simulink model "sampleModel1577"  (R2023a)
settings: Solver=VariableStepAuto  StartTime=0.0  StopTime=10.0  RelTol=1e-3
libraries: hdlsllib x2
settings Model: Creator=user1  LastModifiedBy=user1

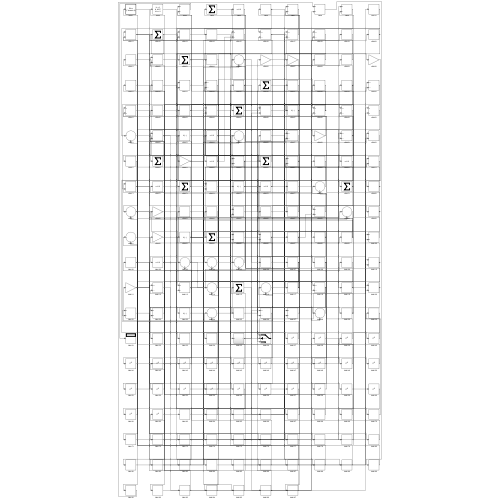
[thumbnail: Simulink's stored preview of the top-level diagram]
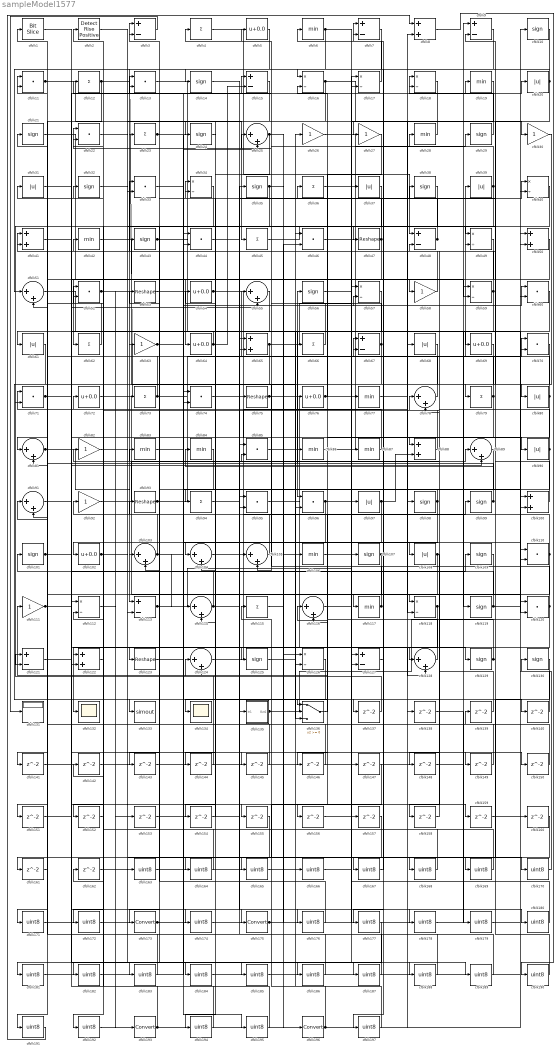
== system sampleModel1577 ==
  cfblk1 : hdlsllib/Logic and Bit Operations/Bit Slice  lidx=7  ridx=0
  cfblk{10,14,21,24,29,32,35,38,43,56,98..99,101,107,109,119,125,129..130} (19 alike) : Signum
  cfblk{8,41,50,65,88,100,122} (7 alike) : Sum
  cfblk{5,54,64,69,72,76,102} (7 alike) : Bias  Bias=0.0  SaturateOnIntegerOverflow=off
  cfblk{25,51,55,78,81,89,91,103..105,114,116,124,128} (14 alike) : Sum  Inputs=|++
  cfblk{6,19,28,42,77,83..84,86..87,106,117} (11 alike) : MinMax
  cfblk{20,31,37,39,61,68,80,90,97,108} (10 alike) : Abs  SaturateOnIntegerOverflow=off
  cfblk{11,13,22,33,44,46,52,60,70..71,74,85,95..96,110,120} (16 alike) : DotProduct  OutDataTypeStr=Inherit: Inherit via internal rule
  cfblk{26..27,30,58,63,82,92,111} (8 alike) : Gain
  cfblk{16..18,34,40,49,57,59,112,118,126} (11 alike) : Product  Inputs=*/  RndMeth=Zero  SaturateOnIntegerOverflow=on
  cfblk{3,7,9,15,48,67,113,121,127} (9 alike) : Sum  Inputs=+-
  cfblk{4,12,23,36,45,62,66,73,79,94,115} (11 alike) : Sum  Inputs=+
  cfblk{47,53,75,93,123} (5 alike) : Reshape
  cfblk131 : Display
  cfblk132 : Scope
  cfblk133 : ToWorkspace  VariableName=simout  SaveFormat=Timeseries  SampleTime=-1
  cfblk134 : Scope
  cfblk135 : Subsystem
      settings: LibrarySourceBlock=|
      | hdlsllib/Ports &
      | Subsystems/Subsystem
  cfblk136 : Switch  SaturateOnIntegerOverflow=off  InputSameDT=off
  cfblk{137..162} (26 alike) : Delay  SampleTime=1
  cfblk{163..172,174,176..192,194..195,197} (31 alike) : DataTypeConversion  OutDataTypeStr=uint8  SaturateOnIntegerOverflow=off  RndMeth=Floor
  cfblk{173,175,193,196} (4 alike) : DataTypeConversion  SaturateOnIntegerOverflow=off  RndMeth=Floor
  cfblk2 : hdlsllib/Logic and Bit Operations/Detect Rise Positive  vinit=0  OutDataTypeStr=boolean
  wires:
  cfblk49/1 -> cfblk64/1
  cfblk54/1 -> cfblk90/1, cfblk96/2
  cfblk62/1 -> cfblk41/1
  cfblk122/1 -> cfblk31/1
  cfblk10/1 -> cfblk51/1
  cfblk115/1 -> cfblk196/1
  cfblk21/1 -> cfblk58/1
  cfblk6/1 -> cfblk113/1, cfblk30/1
  cfblk97/1 -> cfblk111/1, cfblk88/2
  cfblk61/1 -> cfblk133/1
  cfblk47/1 -> cfblk62/1, cfblk13/1, cfblk184/1
  cfblk46/1 -> cfblk79/1
  cfblk75/1 -> cfblk108/1, cfblk128/1
  cfblk128/1 -> cfblk92/1
  cfblk57/1 -> cfblk134/1
  cfblk26/1 -> cfblk29/1
  cfblk29/1 -> cfblk18/1
  cfblk86/1 -> cfblk28/1
  cfblk79/1 -> cfblk32/1, cfblk136/1
  cfblk25/1 -> cfblk104/1, cfblk106/1
  cfblk18/1 -> cfblk113/2
  cfblk72/1 -> cfblk118/1
  cfblk71/1 -> cfblk55/2, cfblk140/1
  cfblk129/1 -> cfblk78/1, cfblk49/2
  cfblk31/1 -> cfblk88/1
  cfblk93/1 -> cfblk39/1, cfblk117/1, cfblk110/2, cfblk3/1, cfblk60/1
  cfblk80/1 -> cfblk55/1, cfblk118/2
  cfblk53/1 -> cfblk96/1
  cfblk95/1 -> cfblk129/1
  cfblk66/1 -> cfblk42/1
  cfblk104/1 -> cfblk99/1
  cfblk44/1 -> cfblk75/1
  cfblk28/1 -> cfblk27/1
  cfblk14/1 -> cfblk135/1(In1)
  cfblk83/1 -> cfblk175/1
  cfblk37/1 -> cfblk173/1
  cfblk12/1 -> cfblk73/1, cfblk161/1
  cfblk117/1 -> cfblk22/1, cfblk12/1
  cfblk101/1 -> cfblk128/2, cfblk174/1
  cfblk13/1 -> cfblk107/1
  cfblk11/1 -> cfblk45/1, cfblk13/2, cfblk66/1
  cfblk125/1 -> cfblk89/1
  cfblk94/1 -> cfblk35/1
  cfblk109/1 -> cfblk124/2
  cfblk99/1 -> cfblk56/1, cfblk21/1, cfblk84/1
  cfblk113/1 -> cfblk57/1, cfblk25/2
  cfblk124/1 -> cfblk19/1
  cfblk68/1 -> cfblk102/1
  cfblk27/1 -> cfblk76/1
  cfblk81/1 -> cfblk103/1, cfblk89/2
  cfblk78/1 -> cfblk67/1
  cfblk51/1 -> cfblk86/1
  cfblk63/1 -> cfblk125/1, cfblk100/2
  cfblk50/1 -> cfblk81/1
  cfblk3/1 -> cfblk131/1
  cfblk4/1 -> cfblk48/1
  cfblk39/1 -> cfblk5/1, cfblk65/2, cfblk192/1
  cfblk112/1 -> cfblk193/1
  cfblk127/1 -> cfblk7/1
  cfblk92/1 -> cfblk70/1
  cfblk30/1 -> cfblk80/1
  cfblk23/1 -> cfblk120/1, cfblk195/1
  cfblk64/1 -> cfblk61/1, cfblk15/2
  cfblk58/1 -> cfblk33/1
  cfblk52/1 -> cfblk105/1, cfblk153/1
  cfblk5/1 -> cfblk33/2
  cfblk103/1 -> cfblk93/1, cfblk57/2, cfblk114/1
  cfblk67/1 -> cfblk104/2, cfblk4/1
  cfblk100/1 -> cfblk38/1
  cfblk73/1 -> cfblk26/1, cfblk11/1
  cfblk17/1 -> cfblk6/1
  cfblk136/1 -> cfblk116/1
  cfblk45/1 -> cfblk47/1
  cfblk76/1 -> cfblk16/2, cfblk189/1
  cfblk85/1 -> cfblk40/1
  cfblk48/1 -> cfblk34/1, cfblk43/1
  cfblk111/1 -> cfblk109/1, cfblk18/2, cfblk155/1
  cfblk7/1 -> cfblk14/1
  cfblk33/1 -> cfblk15/1
  cfblk88/1 -> cfblk52/1
  cfblk96/1 -> cfblk77/1, cfblk152/1
  cfblk20/1 -> cfblk16/1, cfblk69/1
  cfblk43/1 -> cfblk119/1, cfblk3/2
  cfblk77/1 -> cfblk20/1
  cfblk118/1 -> cfblk132/1, cfblk136/3
  cfblk108/1 -> cfblk158/1, cfblk172/1
  cfblk59/1 -> cfblk25/1, cfblk197/1
  cfblk135/1(Out1) -> cfblk50/2, cfblk46/2
  cfblk36/1 -> cfblk120/2
  cfblk98/1 -> cfblk94/1, cfblk136/2
  cfblk107/1 -> cfblk116/2, cfblk191/1
  cfblk70/1 -> cfblk105/2
  cfblk114/1 -> cfblk72/1, cfblk36/1
  cfblk38/1 -> cfblk122/1
  cfblk15/1 -> cfblk24/1
  cfblk42/1 -> cfblk126/2
  cfblk106/1 -> cfblk70/2
  cfblk32/1 -> cfblk49/1
  cfblk40/1 -> cfblk121/2
  cfblk1/1 -> cfblk59/2
  cfblk102/1 -> cfblk159/1, cfblk170/1
  cfblk87/1 -> cfblk71/1
  cfblk16/1 -> cfblk98/1, cfblk23/1, cfblk150/1
  cfblk65/1 -> cfblk71/2, cfblk95/2, cfblk17/2
  cfblk116/1 -> cfblk87/1
  cfblk90/1 -> cfblk41/2, cfblk146/1
  cfblk119/1 -> cfblk100/1, cfblk101/1
  cfblk105/1 -> cfblk54/1
  cfblk35/1 -> cfblk114/2, cfblk166/1
  cfblk110/1 -> cfblk53/1, cfblk123/1
  cfblk34/1 -> cfblk63/1
  cfblk120/1 -> cfblk82/1, cfblk148/1
  cfblk22/1 -> cfblk137/1
  cfblk137/1 -> cfblk121/1
  cfblk139/1 -> cfblk85/2
  cfblk140/1 -> cfblk50/1
  cfblk55/1 -> cfblk141/1
  cfblk141/1 -> cfblk59/1
  cfblk84/1 -> cfblk143/1
  cfblk143/1 -> cfblk103/2
  cfblk89/1 -> cfblk144/1
  cfblk144/1 -> cfblk81/2
  cfblk41/1 -> cfblk145/1
  cfblk145/1 -> cfblk51/2
  cfblk146/1 -> cfblk34/2
  cfblk148/1 -> cfblk48/2
  cfblk82/1 -> cfblk149/1
  cfblk149/1 -> cfblk65/1
  cfblk150/1 -> cfblk67/2
  cfblk69/1 -> cfblk151/1
  cfblk151/1 -> cfblk122/2
  cfblk152/1 -> cfblk52/2
  cfblk153/1 -> cfblk95/1
  cfblk19/1 -> cfblk154/1
  cfblk154/1 -> cfblk124/1
  cfblk60/1 -> cfblk156/1
  cfblk158/1 -> cfblk78/2
  cfblk159/1 -> cfblk40/2
  cfblk161/1 -> cfblk1/1
  cfblk2/1 -> cfblk163/1
  cfblk163/1 -> cfblk97/1
  cfblk126/1 -> cfblk164/1
  cfblk164/1 -> cfblk2/1
  cfblk147/1 -> cfblk165/1
  cfblk165/1 -> cfblk127/2
  cfblk166/1 -> cfblk147/1
  cfblk142/1 -> cfblk167/1
  cfblk167/1 -> cfblk7/2
  cfblk56/1 -> cfblk168/1
  cfblk168/1 -> cfblk142/1
  cfblk130/1 -> cfblk169/1
  cfblk169/1 -> cfblk44/1
  cfblk170/1 -> cfblk130/1
  cfblk157/1 -> cfblk171/1
  cfblk171/1 -> cfblk44/2
  cfblk172/1 -> cfblk157/1
  cfblk173/1 -> cfblk68/1, cfblk176/1
  cfblk174/1 -> cfblk37/1
  cfblk175/1 -> cfblk60/2, cfblk17/1, cfblk126/1
  cfblk176/1 -> cfblk83/1
  cfblk9/1 -> cfblk177/1
  cfblk121/1 -> cfblk178/1
  cfblk178/1 -> cfblk9/1
  cfblk138/1 -> cfblk179/1
  cfblk179/1 -> cfblk9/2
  cfblk74/1 -> cfblk180/1
  cfblk180/1 -> cfblk127/1
  cfblk177/1 -> cfblk181/1
  cfblk181/1 -> cfblk74/1
  cfblk155/1 -> cfblk182/1
  cfblk182/1 -> cfblk74/2
  cfblk160/1 -> cfblk183/1
  cfblk183/1 -> cfblk11/2
  cfblk184/1 -> cfblk160/1
  cfblk162/1 -> cfblk185/1
  cfblk185/1 -> cfblk110/1
  cfblk123/1 -> cfblk186/1
  cfblk186/1 -> cfblk162/1
  cfblk91/1 -> cfblk187/1
  cfblk187/1 -> cfblk85/1
  cfblk156/1 -> cfblk188/1
  cfblk188/1 -> cfblk91/1
  cfblk189/1 -> cfblk91/2
  cfblk8/1 -> cfblk190/1
  cfblk190/1 -> cfblk139/1
  cfblk191/1 -> cfblk8/1
  cfblk192/1 -> cfblk8/2
  cfblk193/1 -> cfblk138/1, cfblk22/2
  cfblk24/1 -> cfblk194/1
  cfblk194/1 -> cfblk112/1
  cfblk195/1 -> cfblk112/2
  cfblk196/1 -> cfblk46/1, cfblk10/1
  cfblk197/1 -> cfblk115/1

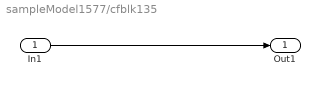
== system sampleModel1577/cfblk135 ==
  In1 : Inport
  Out1 : Outport
  wires:
  In1/1 -> Out1/1
